simulink model "ModellStolVDahlberg"  (R2018a)
settings: Solver=VariableStepAuto  StartTime=0.0  StopTime=10.0  RelTol=1e-3
values from neighbouring files (symbols this model uses):
  c = 250    [SimVDahlbergsKrets.m]
  g = 9.8    [SimVDahlbergsKrets.m]
  k = 25000    [SimVDahlbergsKrets.m]
  m = 5    [SimVDahlbergsKrets.m]
  M = 75    [SimVDahlbergsKrets.m]
settings Model: Creator=Vilmer Dahlberg  LastModifiedBy=Vilmer Dahlberg

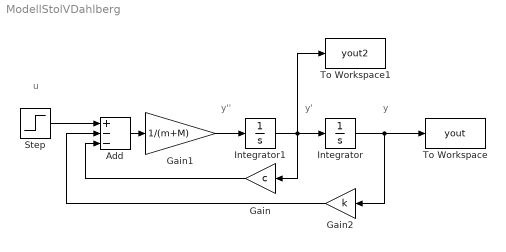
== system ModellStolVDahlberg ==
  note: u
  note: y
  note: y'
  note: y''
  Add : Sum  Inputs=+--
  Gain : Gain  Gain=c
  Gain1 : Gain  Gain=1/(m+M)
  Gain2 : Gain  Gain=k
  Integrator : Integrator  ContinuousStateAttributes='Position'
  Integrator1 : Integrator  ContinuousStateAttributes='Velocity'
  Step : Step  Time=0  After=M*g  SampleTime=0
  To Workspace : ToWorkspace  VariableName=yout  SaveFormat=Timeseries  SampleTime=-1
  To Workspace1 : ToWorkspace  VariableName=yout2  SaveFormat=Timeseries  SampleTime=-1
  wires:
  Integrator1/1 -> Gain/1, Integrator/1, To Workspace1/1
  Integrator/1 -> Gain2/1, To Workspace/1
  Gain2/1 -> Add/2
  Gain/1 -> Add/3
  Add/1 -> Gain1/1
  Gain1/1 -> Integrator1/1
  Step/1 -> Add/1
